simulink model "smdcompare"  (Simulink 9.1)
settings: Solver=ode45  StartTime=0.0  StopTime=10.0  RelTol=1e-3  EnableMultiTasking=on
undefined symbols (not defined in the file or in its folder): b, k, m
settings Model: SuppressorTable=22 serialization::archive 11 0 6 0 0 0 0 0  Creator=Chris Jobling  LastModifiedBy=eechris
settings DataIOCC: LimitDataPoints=on  SignalLoggingSaveFormat=ModelDataLogs
settings OptimizationCC: ExpressionDepthLimit=2147483647
settings DebuggingCC: SolverPrmCheckMsg=warning  FcnCallInpInsideContextMsg=warning  StateNameClashWarn=warning

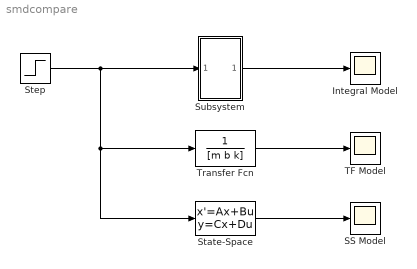
== system smdcompare ==
  Integral Model : Scope
  SS Model : Scope
  State-Space : StateSpace  A=[0 1; -k/m -b/m]  B=[0; 1/m]  C=[1 0]  D=0  InitialCondition=0
  Step : Step  SampleTime=0
  Subsystem : Subsystem
  TF Model : Scope
  Transfer Fcn : TransferFcn  Denominator=[m b k]
  wires:
  Step/1 -> Subsystem/1(In1), Transfer Fcn/1, State-Space/1
  Subsystem/1(Out1) -> Integral Model/1
  Transfer Fcn/1 -> TF Model/1
  State-Space/1 -> SS Model/1

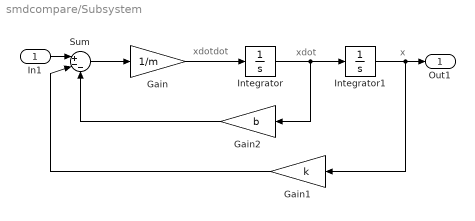
== system smdcompare/Subsystem ==
  note: xdot
  note: xdotdot
  note: x
  In1 : Inport
  Gain : Gain  Gain=1/m
  Gain1 : Gain  Gain=k
  Gain2 : Gain  Gain=b
  Integrator : Integrator
  Integrator1 : Integrator
  Sum : Sum  Inputs=|+--
  Out1 : Outport
  wires:
  Integrator/1 -> Integrator1/1, Gain2/1
  Gain/1 -> Integrator/1
  Integrator1/1 -> Gain1/1, Out1/1
  Gain2/1 -> Sum/3
  Gain1/1 -> Sum/2
  Sum/1 -> Gain/1
  In1/1 -> Sum/1
